simulink model "pump_2"  (R2018b)
settings: Solver=ode45  StartTime=0.0  StopTime=200  MaxStep=5  RelTol=1e-3  EnableMultiTasking=on
undefined symbols (not defined in the file): path_carnot
libraries: carnot x6, simulink x2
settings Model: Creator=drhf  LastModifiedBy=drhf
settings DataIOCC: LimitDataPoints=on  SaveFormat=Array
settings OptimizationCC: ExpressionDepthLimit=2147483647  LifeSpan=inf
settings DebuggingCC: UnderspecifiedInitializationDetection=Classic  MergeDetectMultiDrivingBlocksExec=none  SolverPrmCheckMsg=warning  StateNameClashWarn=warning  SFUnexpectedBacktrackingDiag=warning  SFNoUnconditionalDefaultTransitionDiag=warning  SFExecutionAtInitializationDiag=none
settings HardwareCC: ProdBitPerPointer=32  ProdBitPerSizeT=32  ProdBitPerPtrDiffT=32  ProdLargestAtomicFloat=None  ProdIntDivRoundTo=Undefined  ProdEndianess=Unspecified  ProdWordSize=32  ProdHWDeviceType=32-bit Generic
settings ModelReferenceCC: PropagateSignalLabelsOutOfModel=off
settings SFSimCC: SimUseLocalCustomCode=off
settings RTWCC: RTWUseLocalCustomCode=off
settings CodeAppCC: StateflowObjectComments=on
settings GRTTargetCC: TargetLangStandard=C89/C90 (ANSI)  GeneratePreprocessorConditionals=Disable all  CombineOutputUpdateFcns=off  GRTInterface=on
settings ConfigComp: CovMetricSettings=dw  CovHtmlReporting=on  CovSaveCumulativeToWorkspaceVar=on  CovSaveSingleToWorkspaceVar=on  CovExternalEMLEnable=off

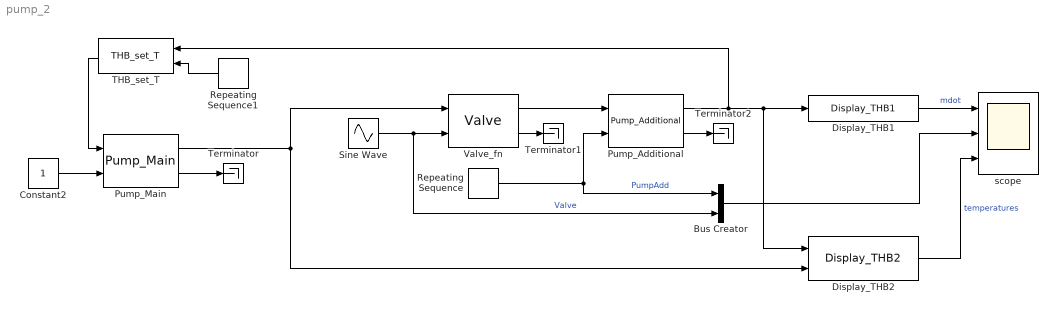
== system pump_2 ==
  Bus Creator : BusCreator  Inputs=2
  Constant2 : Constant
  Display_THB1 : carnot/Outputs/Display_THB1  t=off  m=on  p=off  id=off  mix=off  d=off
  Display_THB2 : carnot/Outputs/Display_THB2  t=on  m=off  p=off  id=off  mix=off  d=off
  Pump_Additional : carnot/Hydraulics/Pump_Additional  Tini=20  PathName=fullfile(path_carnot('libsl'), 'Hydraulics', 'Pump_Main', 'parameter_set')  FileName='Pump5m.mat'  userPath=off  userParam=off  a0=50000  a1=-45000  a2=0  dia=0.025  UA=1  mcp=4182  e0=35  e1=22.5  e2=-8.1
  Pump_Main : carnot/Hydraulics/Pump_Main  Tini=20  p0=3e5  IDpreset=pressure drop  fluid=Water  mix=0  mix2=0  mix3=0  t1=1  PathName=fullfile(path_carnot('libsl'), 'Hydraulics', 'Pump_Main', 'parameter_set')  FileName='Pump6m.mat'  userPath=off  userParam=off  a0=60000  a1=-43200  a2=0  dia=0.025  UA=1  mcp=4182  e0=50  e1=28.8  e2=-10.368
  Repeating Sequence : simulink/Sources/Repeating Sequence  rep_seq_t=[0 90 100 200]  rep_seq_y=[0 0 1 1]
  Repeating Sequence1 : simulink/Sources/Repeating Sequence  rep_seq_t=[ 0 120 120+eps(120) 200]  rep_seq_y=[ 20 20 40+0*eps(120) 40]
  Sine Wave : Sin  Amplitude=0.6  Bias=0.5  Frequency=1/20  SampleTime=0
  THB_set_T : carnot/Source/Simple/THB_set_T
  Terminator : Terminator
  Terminator1 : Terminator
  Terminator2 : Terminator
  Valve_fn : carnot/Hydraulics/Valve  vtyp=linear  psi_0=0.04  kvs=0.9  dt_V=30
  scope : Scope  NumInputPorts=3
  wires:
  Constant2/1 -> Pump_Main/2
  Pump_Main/2 -> Terminator/1
  Sine Wave/1 -> Bus Creator/2, Valve_fn/2  "Valve"
  Pump_Main/1 -> Valve_fn/1, Display_THB2/2
  Display_THB1/1 -> scope/1  "mdot"
  Valve_fn/1 -> Pump_Additional/1
  Repeating Sequence/1 -> Pump_Additional/2, Bus Creator/1  "PumpAdd"
  Pump_Additional/2 -> Terminator2/1
  Pump_Additional/1 -> THB_set_T/1, Display_THB1/1, Display_THB2/1
  THB_set_T/1 -> Pump_Main/1
  Repeating Sequence1/1 -> THB_set_T/2
  Bus Creator/1 -> scope/2
  Display_THB2/1 -> scope/3  "temperatures"
  Valve_fn/2 -> Terminator1/1
